simulink model "fcs_archi"  (R2023b)
settings: Solver=FixedStepAuto  StartTime=0.0  StopTime=10.0  FixedStep=5e-5  RelTol=1e-3
InitFcn:
  | addpath('c\');
  | addpath('enums\');
values from neighbouring files (symbols this model uses):
  Climb_Alt = 50.0    [fcs_spec.sldd]
  density_of_air = 1.2    [fcs_spec.sldd]
  f_Baro_Alt = 50.0    [fcs_spec.sldd]
  f_fidr = 400.0    [fcs_spec.sldd]
  f_GPS = 10.0    [fcs_spec.sldd]
  f_IMU = 800.0    [fcs_spec.sldd]
  f_inner_loop = 400.0    [fcs_spec.sldd]
  f_Mag = 50.0    [fcs_spec.sldd]
  f_mission_manager = 50.0    [fcs_spec.sldd]
  f_outer_loop = 50.0    [fcs_spec.sldd]
  f_Pitot = 50.0    [fcs_spec.sldd]
  f_sensor_acquisition = 400.0    [fcs_spec.sldd]
  g = 9.8    [fcs_spec.sldd]
  Pitch_Angle_Max = 0.4363    [fcs_spec.sldd]
  Pitch_Angle_Min = -0.261799    [fcs_spec.sldd]
  Pitch_Rate_Max = 1.05    [fcs_spec.sldd]
  Roll_Angle_Max = 1.15    [fcs_spec.sldd]
  Roll_Rate_Max = 1.57    [fcs_spec.sldd]
  Takeoff_Alt = 2.0    [fcs_spec.sldd]
  Takeoff_Spd = 50.0    [fcs_spec.sldd]
  Yaw_Rate_Max = 0.52    [fcs_spec.sldd]
undefined symbols (not defined in the file or in its folder): DiscIntNeverNeededParam, Sensor_Mode
libraries: dspfdesign x5, simulink x3, sharedtransform x1
(part 1 of 2)
settings Model: DataDictionary=fcs_spec.sldd  Creator=Aniket  LastModifiedBy=Aniket
settings SFSimCC: SimUserIncludeDirs=.\c
settings SFSimCC: SimCustomHeaderCode=|
  | #include "attitude_controller.h"
  | #include "pos_alt_controller.h"
settings SFSimCC: SimUserSources=|
  | attitude_controller.c
  | pos_alt_controller.c
settings ConfigComp: DVTestSuiteOptimization=Auto  DVDetectOutOfBounds=on  DVModelReferenceHarness=on  DVHarnessSource=Signal Editor  DVRebuildModelRepresentation=IfChangeIsDetected

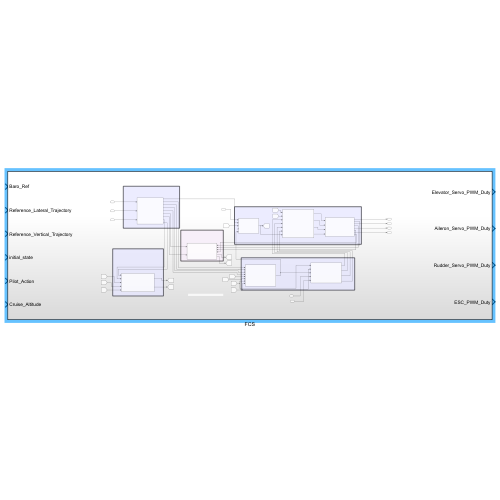
[thumbnail: Simulink's stored preview of the top-level diagram]
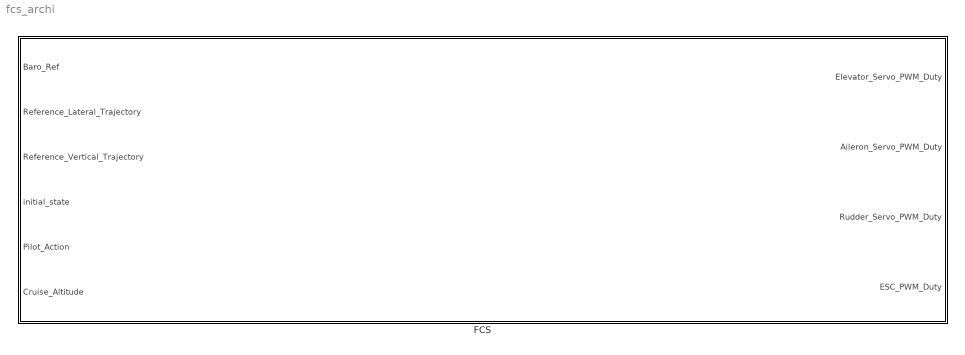
== system fcs_archi ==
  FCS : Subsystem

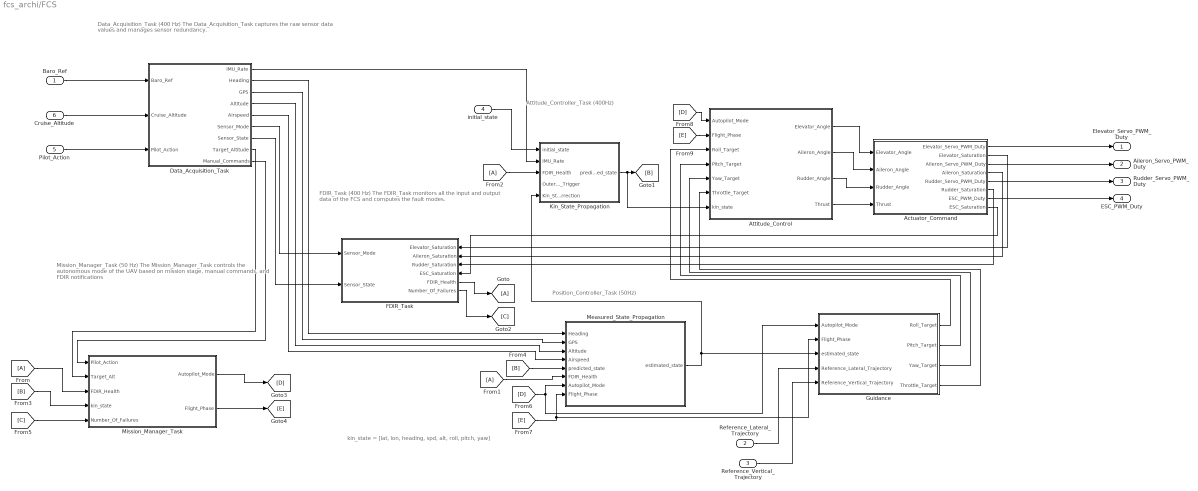
== system fcs_archi/FCS ==
  note: kin_state = [lat, lon, heading, spd, alt, roll, pitch, yaw]
  note: Mission_Manager_Task (50 Hz)
      | The Mission_Manager_Task controls the autonomous mode
      | of the UAV based on mission stage, manual commands, and
      | FDIR notifications
  note: Attitude_Controller_Task (400Hz)
  note: FDIR_Task (400 Hz)
      | The FDIR_Task monitors all the input
      | and output data of the FCS and computes the fault
      | modes.
  note: Data_Acquisition_Task (400 Hz)
      | The Data_Acquisition_Task captures the raw sensor data values
      | and manages sensor redundancy.
  note: Position_Controller_Task (50Hz)
  Baro_Ref : Inport
  Reference_Lateral_Trajectory : Inport  Port=2
  Reference_Vertical_Trajectory : Inport  Port=3
  initial_state : Inport  Port=4
  Pilot_Action : Inport  Port=5
  Cruise_Altitude : Inport  Port=6
  Actuator_Command : Subsystem
  Attitude_Control : Subsystem
  Data_Acquisition_Task : Subsystem
  FDIR_Task : Subsystem
      settings: PortSchema="{\"entries\":[{\"content\":{\"sides\":[{\"content\":{\"connectorIds\":[\"In1\",\"In2\"]},\"type\":\"ConnectorPlacement.EquallySpacedRectSide\",\"uuid\":\"991e8061-6223-401d-b3d8-a02ac305caf5\"},{\"content\":{\"connectorIds\":[\"In3\",\"In4\",\"In5\",\"In6\",\"Out1\",\"Out2\"],\"side\":\"RIGHT\"},\"type\":\"ConnectorPlacement.EquallySpacedRectSide\",\"uuid\":\"39839a1c-9529-4bba-bfe7-212855812bb8\"},{\"content\":{\"side\":\"TOP\"},\"type\":\"ConnectorPlacement.EquallySpacedRectSide\",\"uuid\":\"1450207f-9818-4db6-97f8-8e2891081434\"}]},\"type\":\"ConnectorPlacement.EquallySpacedConnector\",\"uuid\":\"30fba5ee-2c18-47f5-b9c2-5959a4a20b0d\"}],\"packageUris\":[\"http://schema.mathworks.com/mf0/Connector/R2020b\"],\"version\":\"1.0\"}"
  From : From
  From1 : From
  From2 : From
  Goto : Goto
  Guidance : Subsystem
  Kin_State_Propagation : Subsystem
  Measured_State_Propagation : Subsystem
  Mission_Manager_Task : Subsystem
  Elevator_Servo_PWM_Duty : Outport
  Aileron_Servo_PWM_Duty : Outport  Port=2
  Rudder_Servo_PWM_Duty : Outport  Port=3
  ESC_PWM_Duty : Outport  Port=4
  wires:
  Reference_Vertical_Trajectory/1 -> Guidance/5(Reference_Vertical_Trajectory)
  Data_Acquisition_Task/4(Altitude) -> Measured_State_Propagation/3(Altitude)
  Measured_State_Propagation/1(estimated_state) -> Kin_State_Propagation/5(Kin_State_correction), Guidance/3(estimated_state)
  Data_Acquisition_Task/6(Sensor_Mode) -> FDIR_Task/1(Sensor_Mode)
  Kin_State_Propagation/1(predicted_state) -> [B], Attitude_Control/7(kin_state)
  Data_Acquisition_Task/2(Heading) -> Measured_State_Propagation/1(Heading)
  Data_Acquisition_Task/3(GPS) -> Measured_State_Propagation/2(GPS)
  Actuator_Command/3(Aileron_Servo_PWM_Duty) -> Aileron_Servo_PWM_Duty/1
  Data_Acquisition_Task/7(Sensor_State) -> FDIR_Task/2(Sensor_State)
  Guidance/3(Yaw_Target) -> Attitude_Control/5(Yaw_Target)
  Data_Acquisition_Task/5(Airspeed) -> Measured_State_Propagation/4(Airspeed)
  Actuator_Command/6(Rudder_Saturation) -> FDIR_Task/5(Rudder_Saturation)
  Actuator_Command/2(Elevator_Saturation) -> FDIR_Task/3(Elevator_Saturation)
  Guidance/4(Throttle_Target) -> Attitude_Control/6(Throttle_Target)
  Data_Acquisition_Task/1(IMU_Rate) -> Kin_State_Propagation/2(IMU_Rate)
  Reference_Lateral_Trajectory/1 -> Guidance/4(Reference_Lateral_Trajectory)
  Guidance/1(Roll_Target) -> Attitude_Control/3(Roll_Target)
  Actuator_Command/5(Rudder_Servo_PWM_Duty) -> Rudder_Servo_PWM_Duty/1
  Guidance/2(Pitch_Target) -> Attitude_Control/4(Pitch_Target)
  Attitude_Control/3(Rudder_Angle) -> Actuator_Command/3(Rudder_Angle)
  Actuator_Command/4(Aileron_Saturation) -> FDIR_Task/4(Aileron_Saturation)
  Attitude_Control/1(Elevator_Angle) -> Actuator_Command/1(Elevator_Angle)
  Attitude_Control/4(Thrust) -> Actuator_Command/4(Thrust)
  Attitude_Control/2(Aileron_Angle) -> Actuator_Command/2(Aileron_Angle)
  Actuator_Command/8(ESC_Saturation) -> FDIR_Task/6(ESC_Saturation)
  Baro_Ref/1 -> Data_Acquisition_Task/1(Baro_Ref)
  Actuator_Command/1(Elevator_Servo_PWM_Duty) -> Elevator_Servo_PWM_Duty/1
  Actuator_Command/7(ESC_PWM_Duty) -> ESC_PWM_Duty/1
  initial_state/1 -> Kin_State_Propagation/1(initial_state)
  FDIR_Task/1(FDIR_Health) -> Goto/1
  From/1 -> Mission_Manager_Task/3(FDIR_Health)
  From1/1 -> Measured_State_Propagation/6(FDIR_Health)
  From2/1 -> Kin_State_Propagation/3(FDIR_Health)
  [B] -> Mission_Manager_Task/4(kin_state)
  [B] -> Measured_State_Propagation/5(predicted_state)
  Pilot_Action/1 -> Data_Acquisition_Task/3(Pilot_Action)
  FDIR_Task/2(Number_Of_Failures) -> [C]
  [C] -> Mission_Manager_Task/5(Number_Of_Failures)
  Cruise_Altitude/1 -> Data_Acquisition_Task/2(Cruise_Altitude)
  Mission_Manager_Task/1(Autopilot_Mode) -> [D]
  Mission_Manager_Task/2(Flight_Phase) -> [E]
  [D] -> Attitude_Control/1(Autopilot_Mode)
  [E] -> Attitude_Control/2(Flight_Phase)
  Data_Acquisition_Task/9(Manual_Commands) -> Mission_Manager_Task/1(Pilot_Action)
  Data_Acquisition_Task/8(Target_Altitude) -> Mission_Manager_Task/2(Target_Alt)
  [D] -> Measured_State_Propagation/7(Autopilot_Mode), Guidance/1(Autopilot_Mode)
  [E] -> Measured_State_Propagation/8(Flight_Phase), Guidance/2(Flight_Phase)

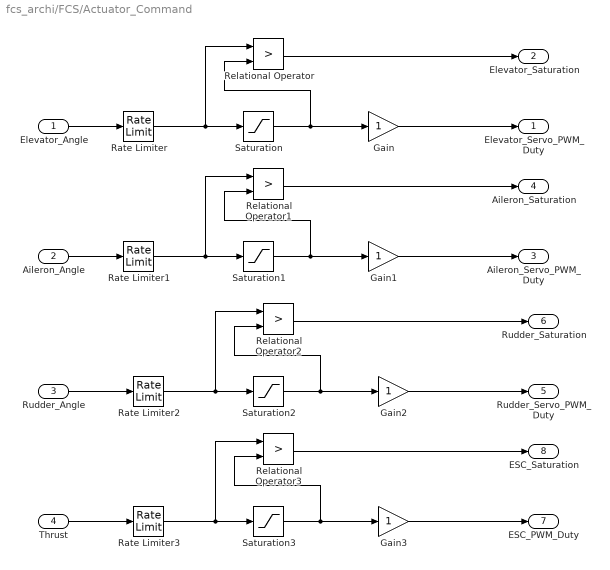
== system fcs_archi/FCS/Actuator_Command ==
  Elevator_Angle : Inport
  Aileron_Angle : Inport  Port=2
  Rudder_Angle : Inport  Port=3
  Thrust : Inport  Port=4
  Gain{,1..3} (4 alike) : Gain
  Rate Limiter{,1..3} (4 alike) : RateLimiter  SampleTimeMode=inherited
  Relational Operator{,1..3} (4 alike) : RelationalOperator  Operator=>  OutDataTypeStr=boolean  RndMeth=Simplest  InputSameDT=off
  Saturation{,1..3} (4 alike) : Saturate
  Elevator_Servo_PWM_Duty : Outport
  Elevator_Saturation : Outport  Port=2
  Aileron_Servo_PWM_Duty : Outport  Port=3
  Aileron_Saturation : Outport  Port=4
  Rudder_Servo_PWM_Duty : Outport  Port=5
  Rudder_Saturation : Outport  Port=6
  ESC_PWM_Duty : Outport  Port=7
  ESC_Saturation : Outport  Port=8
  wires:
  Elevator_Angle/1 -> Rate Limiter/1
  Rate Limiter/1 -> Relational Operator/1, Saturation/1
  Saturation/1 -> Relational Operator/2, Gain/1
  Gain/1 -> Elevator_Servo_PWM_Duty/1
  Relational Operator/1 -> Elevator_Saturation/1
  Relational Operator1/1 -> Aileron_Saturation/1
  Rate Limiter1/1 -> Relational Operator1/1, Saturation1/1
  Gain1/1 -> Aileron_Servo_PWM_Duty/1
  Saturation1/1 -> Relational Operator1/2, Gain1/1
  Aileron_Angle/1 -> Rate Limiter1/1
  Relational Operator2/1 -> Rudder_Saturation/1
  Saturation3/1 -> Relational Operator3/2, Gain3/1
  Rate Limiter3/1 -> Relational Operator3/1, Saturation3/1
  Relational Operator3/1 -> ESC_Saturation/1
  Gain3/1 -> ESC_PWM_Duty/1
  Rate Limiter2/1 -> Relational Operator2/1, Saturation2/1
  Gain2/1 -> Rudder_Servo_PWM_Duty/1
  Saturation2/1 -> Relational Operator2/2, Gain2/1
  Rudder_Angle/1 -> Rate Limiter2/1
  Thrust/1 -> Rate Limiter3/1

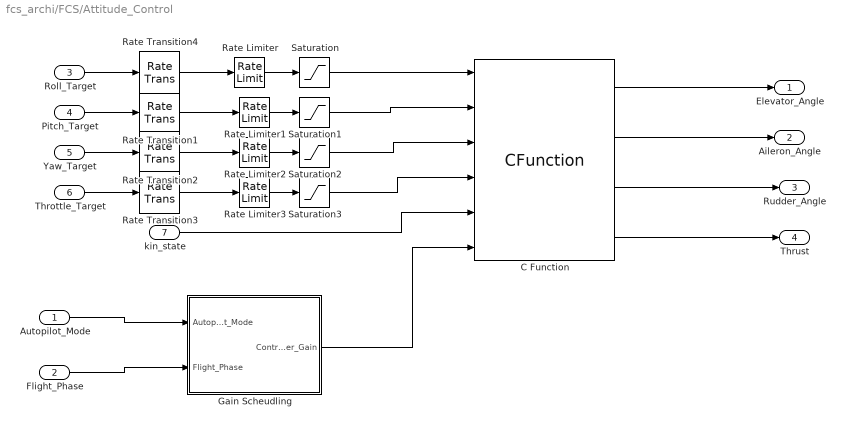
== system fcs_archi/FCS/Attitude_Control ==
  Autopilot_Mode : Inport
  Flight_Phase : Inport  Port=2
  Roll_Target : Inport  Port=3
  Pitch_Target : Inport  Port=4
  Yaw_Target : Inport  Port=5
  Throttle_Target : Inport  Port=6
  kin_state : Inport  Port=7
  C Function : CFunction  OutputCode=compute(Gain, Roll_Target, Pitch_Target, Yaw_Target, Throttle_Target, kin_state, &Elevator_Angle, &Aileron_Angle, &Rudder_Angle, &Thrust);
  Gain Scheudling : Subsystem  TreatAsAtomicUnit=on
  Rate Limiter{,1..3} (4 alike) : RateLimiter  SampleTimeMode=inherited
  Rate Transition{1..4} (4 alike) : RateTransition  OutPortSampleTime=1/f_inner_loop
  Saturation{,1..3} (4 alike) : Saturate
  Elevator_Angle : Outport
  Aileron_Angle : Outport  Port=2
  Rudder_Angle : Outport  Port=3
  Thrust : Outport  Port=4
  wires:
  Roll_Target/1 -> Rate Transition4/1
  Pitch_Target/1 -> Rate Transition1/1
  Yaw_Target/1 -> Rate Transition2/1
  Throttle_Target/1 -> Rate Transition3/1
  Rate Limiter/1 -> Saturation/1
  Saturation/1 -> C Function/1
  Rate Limiter1/1 -> Saturation1/1
  Saturation1/1 -> C Function/2
  Rate Limiter2/1 -> Saturation2/1
  Saturation2/1 -> C Function/3
  Rate Limiter3/1 -> Saturation3/1
  Saturation3/1 -> C Function/4
  kin_state/1 -> C Function/5
  C Function/1 -> Elevator_Angle/1
  C Function/2 -> Aileron_Angle/1
  C Function/3 -> Rudder_Angle/1
  C Function/4 -> Thrust/1
  Rate Transition4/1 -> Rate Limiter/1
  Rate Transition1/1 -> Rate Limiter1/1
  Rate Transition3/1 -> Rate Limiter3/1
  Rate Transition2/1 -> Rate Limiter2/1
  Autopilot_Mode/1 -> Gain Scheudling/1(Autopilot_Mode)
  Flight_Phase/1 -> Gain Scheudling/2(Flight_Phase)
  Gain Scheudling/1(Controller_Gain) -> C Function/6

== system fcs_archi/FCS/Data_Acquisition_Task ==
  Baro_Ref : Inport
  Cruise_Altitude : Inport  Port=2
  Pilot_Action : Inport  Port=3
  Data_Acquisition : Subsystem
  Measurement : Subsystem
  IMU_Rate : Outport
  Heading : Outport  Port=2
  GPS : Outport  Port=3
  Altitude : Outport  Port=4
  Airspeed : Outport  Port=5
  Sensor_Mode : Outport  Port=6
  Sensor_State : Outport  Port=7
  Target_Altitude : Outport  Port=8
  Manual_Commands : Outport  Port=9
  wires:
  Data_Acquisition/1(IMU_Mean) -> Measurement/1(IMU_Mean)
  Data_Acquisition/2(Mag_Mean) -> Measurement/2(Mag_Mean)
  Data_Acquisition/3(GPS_Mean) -> Measurement/3(GPS_Mean)
  Data_Acquisition/4(Baro_Alt_Mean) -> Measurement/4(Baro_Alt_Mean)
  Data_Acquisition/5(Pitot_Mean) -> Measurement/5(Pitot_Mean)
  Data_Acquisition/6(Mode) -> Sensor_Mode/1
  Data_Acquisition/7(Sensor_State) -> Sensor_State/1
  Baro_Ref/1 -> Measurement/6(Baro_Ref)
  Measurement/1(IMU_Rate) -> IMU_Rate/1
  Measurement/3(GPS) -> GPS/1
  Measurement/2(Heading) -> Heading/1
  Measurement/5(Airspeed) -> Airspeed/1
  Measurement/4(Altitude) -> Altitude/1
  Cruise_Altitude/1 -> Data_Acquisition/1(Cruise_Altitude_Raw)
  Pilot_Action/1 -> Data_Acquisition/2(Pilot_Action_Raw)
  Data_Acquisition/8(Cruise_Altitude) -> Target_Altitude/1
  Data_Acquisition/9(Pilot_Action) -> Manual_Commands/1

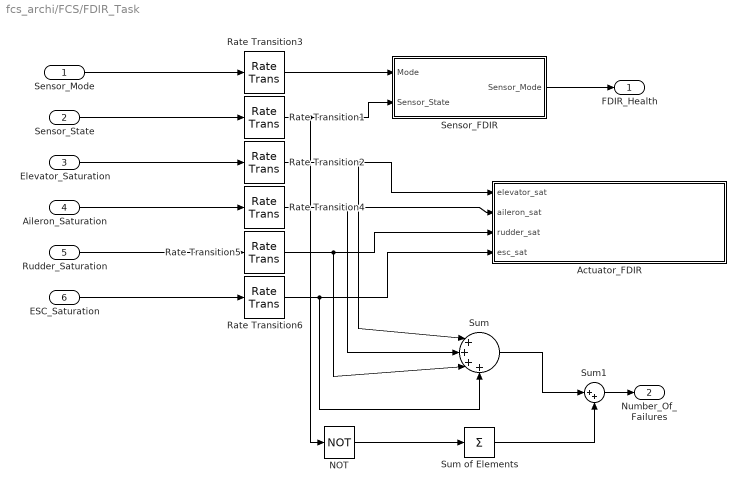
== system fcs_archi/FCS/FDIR_Task ==
  Sensor_Mode : Inport  OutDataTypeStr=Enum: Sensor_Mode
  Sensor_State : Inport  Port=2
  Elevator_Saturation : Inport  Port=3
  Aileron_Saturation : Inport  Port=4
  Rudder_Saturation : Inport  Port=5
  ESC_Saturation : Inport  Port=6
  Actuator_FDIR : MATLAB Function  TreatAsAtomicUnit=on
  NOT : Logic  Operator=NOT  IconShape=distinctive  AllPortsSameDT=off  OutDataTypeStr=boolean
  Rate Transition{1..6} (6 alike) : RateTransition  OutPortSampleTime=1/f_fidr
  Sensor_FDIR : Subsystem
  Sum : Sum  Inputs=|++++
  Sum of Elements : Sum  Inputs=+
  Sum1 : Sum  Inputs=|++
  FDIR_Health : Outport
  Number_Of_Failures : Outport  Port=2
  wires:
  Sensor_Mode/1 -> Rate Transition3/1
  Sensor_State/1 -> Rate Transition1/1
  Sensor_FDIR/1(Sensor_Mode) -> FDIR_Health/1
  Rate Transition3/1 -> Sensor_FDIR/1(Mode)
  Rate Transition1/1 -> NOT/1, Sensor_FDIR/2(Sensor_State)
  Elevator_Saturation/1 -> Rate Transition2/1
  Aileron_Saturation/1 -> Rate Transition4/1
  Rudder_Saturation/1 -> Rate Transition5/1
  ESC_Saturation/1 -> Rate Transition6/1
  Rate Transition2/1 -> Actuator_FDIR/1(elevator_sat), Sum/1
  Rate Transition4/1 -> Actuator_FDIR/2(aileron_sat), Sum/2
  Rate Transition5/1 -> Sum/3, Actuator_FDIR/3(rudder_sat)
  Rate Transition6/1 -> Actuator_FDIR/4(esc_sat), Sum/4
  NOT/1 -> Sum of Elements/1
  Sum/1 -> Sum1/1
  Sum of Elements/1 -> Sum1/2
  Sum1/1 -> Number_Of_Failures/1

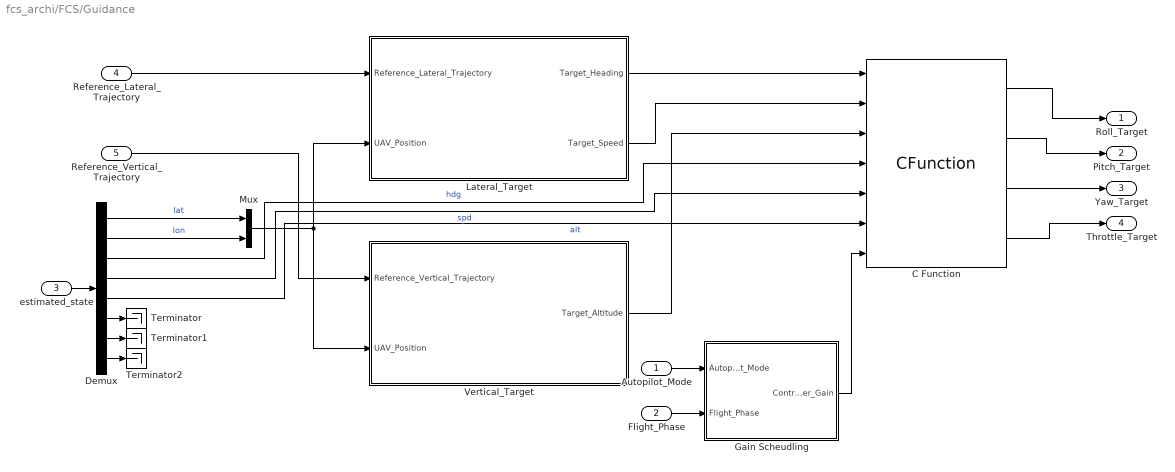
== system fcs_archi/FCS/Guidance ==
  Autopilot_Mode : Inport
  Flight_Phase : Inport  Port=2
  estimated_state : Inport  Port=3
  Reference_Lateral_Trajectory : Inport  Port=4
  Reference_Vertical_Trajectory : Inport  Port=5
  C Function : CFunction  OutputCode=compute_targets(Gain, Target_Hdg, Target_Spd, Target_Alt, Estimated_Hdg, Estimated_Spd, Estimated_Alt, &Roll_Target, &Pitch_Target, &Yaw_Target, &Throttle_Target);
  Demux : Demux  Outputs=8
  Gain Scheudling : Subsystem  TreatAsAtomicUnit=on
  Lateral_Target : Subsystem
  Mux : Mux  Inputs=2
  Terminator : Terminator
  Terminator1 : Terminator
  Terminator2 : Terminator
  Vertical_Target : Subsystem
  Roll_Target : Outport
  Pitch_Target : Outport  Port=2
  Yaw_Target : Outport  Port=3
  Throttle_Target : Outport  Port=4
  wires:
  Reference_Lateral_Trajectory/1 -> Lateral_Target/1(Reference_Lateral_Trajectory)
  estimated_state/1 -> Demux/1
  Demux/1 -> Mux/1  "lat"
  Demux/2 -> Mux/2  "lon"
  Mux/1 -> Vertical_Target/2(UAV_Position), Lateral_Target/2(UAV_Position)
  Reference_Vertical_Trajectory/1 -> Vertical_Target/1(Reference_Vertical_Trajectory)
  Lateral_Target/1(Target_Heading) -> C Function/1
  Lateral_Target/2(Target_Speed) -> C Function/2
  Vertical_Target/1(Target_Altitude) -> C Function/3
  Demux/3 -> C Function/4  "hdg"
  Demux/4 -> C Function/5  "spd"
  Demux/5 -> C Function/6  "alt"
  Demux/6 -> Terminator/1
  Demux/7 -> Terminator1/1
  Demux/8 -> Terminator2/1
  C Function/1 -> Roll_Target/1
  C Function/2 -> Pitch_Target/1
  C Function/3 -> Yaw_Target/1
  C Function/4 -> Throttle_Target/1
  Flight_Phase/1 -> Gain Scheudling/2(Flight_Phase)
  Autopilot_Mode/1 -> Gain Scheudling/1(Autopilot_Mode)
  Gain Scheudling/1(Controller_Gain) -> C Function/7

== system fcs_archi/FCS/Kin_State_Propagation ==
  initial_state : Inport
  IMU_Rate : Inport  Port=2
  FDIR_Health : Inport  Port=3
  Outer_Loop_Trigger : Inport  Port=4
  Kin_State_correction : Inport  Port=5
  "Kin_State2UAV_State " : Subsystem
  Kinematics_Propagator : Subsystem
  Mux : Mux  Inputs=8
  Rate Transition1 : RateTransition  OutPortSampleTime=1/f_inner_loop
  Rate Transition3 : RateTransition  OutPortSampleTime=1/f_inner_loop
  Rate Transition4 : RateTransition  OutPortSampleTime=1/f_inner_loop
  Switch : Switch  Criteria=u2 > Threshold  SaturateOnIntegerOverflow=off  InputSameDT=off
  UAV kinematics : Subsystem
  predicted_state : Outport
  wires:
  Kinematics_Propagator/1(dstate) -> UAV kinematics/2(dstate)
  UAV kinematics/1(state) -> Kinematics_Propagator/3(prev_state), "Kin_State2UAV_State "/1(state)  "Prediction"
  "Kin_State2UAV_State "/7(pitch) -> Mux/7
  "Kin_State2UAV_State "/2(lon) -> Mux/2
  "Kin_State2UAV_State "/4(speed) -> Mux/4
  "Kin_State2UAV_State "/3(heading) -> Mux/3
  "Kin_State2UAV_State "/5(altitude) -> Mux/5
  "Kin_State2UAV_State "/8(yaw) -> Mux/8
  FDIR_Health/1 -> Rate Transition1/1
  "Kin_State2UAV_State "/1(lat) -> Mux/1
  "Kin_State2UAV_State "/6(roll) -> Mux/6
  IMU_Rate/1 -> Rate Transition3/1
  Mux/1 -> Switch/3
  Kin_State_correction/1 -> Rate Transition4/1
  Rate Transition3/1 -> Kinematics_Propagator/1(IMU_Rate)
  Rate Transition1/1 -> Kinematics_Propagator/2(FDIR_Health)
  initial_state/1 -> UAV kinematics/1(initial_state)
  Outer_Loop_Trigger/1 -> Switch/2
  Rate Transition4/1 -> Switch/1
  Switch/1 -> predicted_state/1

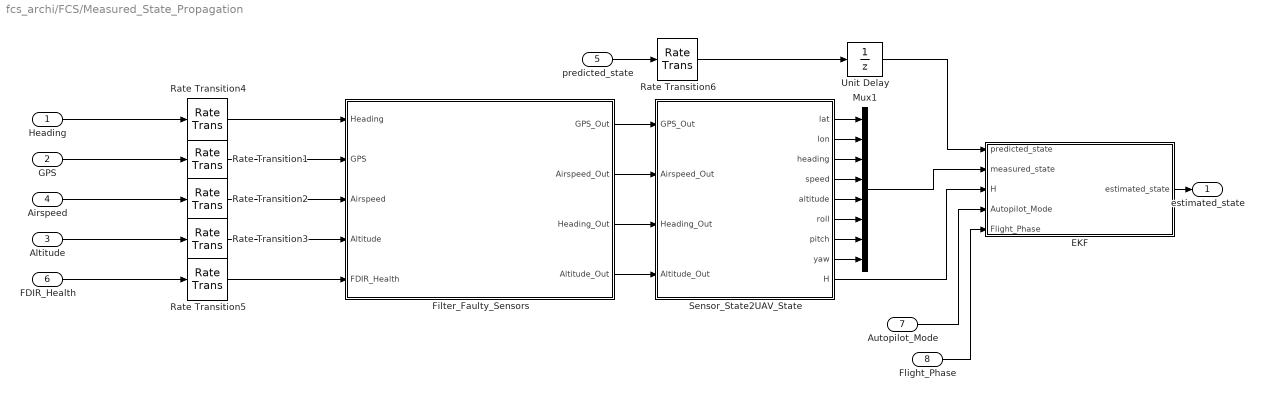
== system fcs_archi/FCS/Measured_State_Propagation ==
  Heading : Inport
  GPS : Inport  Port=2
  Altitude : Inport  Port=3
  Airspeed : Inport  Port=4
  predicted_state : Inport  Port=5
  FDIR_Health : Inport  Port=6
  Autopilot_Mode : Inport  Port=7
  Flight_Phase : Inport  Port=8
  EKF : Subsystem
  Filter_Faulty_Sensors : Subsystem
  Mux1 : Mux  Inputs=8
  Rate Transition{1..5} (5 alike) : RateTransition  OutPortSampleTime=1/f_outer_loop
  Rate Transition6 : RateTransition  OutPortSampleTime=1/f_inner_loop
  Sensor_State2UAV_State : Subsystem
  Unit Delay : UnitDelay  SampleTime=-1  HasFrameUpgradeWarning=on
  estimated_state : Outport
  wires:
  FDIR_Health/1 -> Rate Transition5/1
  Mux1/1 -> EKF/2(measured_state)
  Sensor_State2UAV_State/2(lon) -> Mux1/2
  Airspeed/1 -> Rate Transition2/1
  Sensor_State2UAV_State/1(lat) -> Mux1/1
  predicted_state/1 -> Rate Transition6/1
  EKF/1(estimated_state) -> estimated_state/1
  Filter_Faulty_Sensors/1(GPS_Out) -> Sensor_State2UAV_State/1(GPS_Out)
  Filter_Faulty_Sensors/2(Airspeed_Out) -> Sensor_State2UAV_State/2(Airspeed_Out)
  Filter_Faulty_Sensors/4(Altitude_Out) -> Sensor_State2UAV_State/4(Altitude_Out)
  Altitude/1 -> Rate Transition3/1
  Filter_Faulty_Sensors/3(Heading_Out) -> Sensor_State2UAV_State/3(Heading_Out)
  Sensor_State2UAV_State/9(H) -> EKF/3(H)
  GPS/1 -> Rate Transition1/1
  Heading/1 -> Rate Transition4/1
  Sensor_State2UAV_State/3(heading) -> Mux1/3
  Sensor_State2UAV_State/4(speed) -> Mux1/4
  Sensor_State2UAV_State/5(altitude) -> Mux1/5
  Sensor_State2UAV_State/6(roll) -> Mux1/6
  Sensor_State2UAV_State/7(pitch) -> Mux1/7
  Sensor_State2UAV_State/8(yaw) -> Mux1/8
  Rate Transition4/1 -> Filter_Faulty_Sensors/1(Heading)
  Rate Transition1/1 -> Filter_Faulty_Sensors/2(GPS)
  Rate Transition2/1 -> Filter_Faulty_Sensors/3(Airspeed)
  Rate Transition5/1 -> Filter_Faulty_Sensors/5(FDIR_Health)
  Rate Transition3/1 -> Filter_Faulty_Sensors/4(Altitude)
  Rate Transition6/1 -> Unit Delay/1
  Unit Delay/1 -> EKF/1(predicted_state)
  Autopilot_Mode/1 -> EKF/4(Autopilot_Mode)
  Flight_Phase/1 -> EKF/5(Flight_Phase)

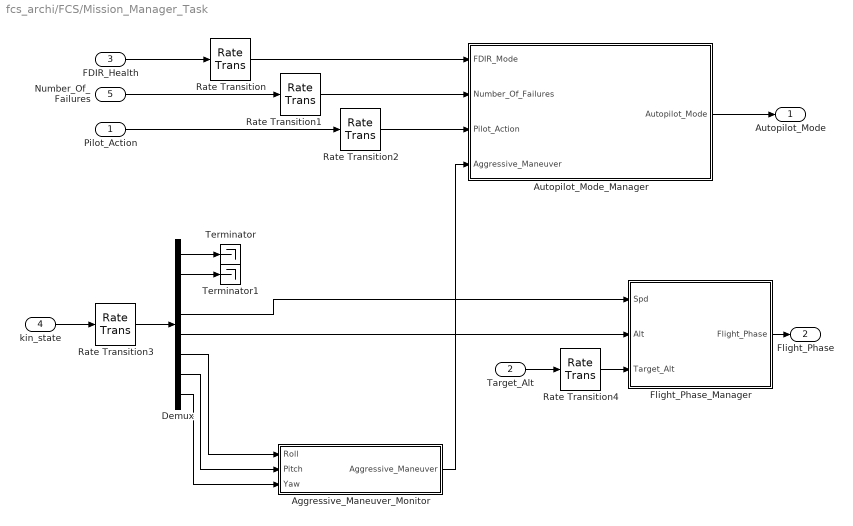
== system fcs_archi/FCS/Mission_Manager_Task ==
  Pilot_Action : Inport
  Target_Alt : Inport  Port=2
  FDIR_Health : Inport  Port=3
  kin_state : Inport  Port=4
  Number_Of_Failures : Inport  Port=5
  Aggressive_Maneuver_Monitor : Subsystem
  Autopilot_Mode_Manager : Stateflow chart  TreatAsAtomicUnit=on
  Demux : Demux  Outputs=8
  Flight_Phase_Manager : Stateflow chart  TreatAsAtomicUnit=on
  Rate Transition{,1..4} (5 alike) : RateTransition  OutPortSampleTime=1/f_mission_manager
  Terminator : Terminator
  Terminator1 : Terminator
  Autopilot_Mode : Outport
  Flight_Phase : Outport  Port=2
  wires:
  kin_state/1 -> Rate Transition3/1
  Target_Alt/1 -> Rate Transition4/1
  Demux/4 -> Flight_Phase_Manager/1(Spd)
  Demux/5 -> Flight_Phase_Manager/2(Alt)
  Demux/1 -> Terminator/1
  Demux/2 -> Terminator1/1
  Demux/6 -> Aggressive_Maneuver_Monitor/1(Roll)
  Demux/7 -> Aggressive_Maneuver_Monitor/2(Pitch)
  Demux/8 -> Aggressive_Maneuver_Monitor/3(Yaw)
  Number_Of_Failures/1 -> Rate Transition1/1
  FDIR_Health/1 -> Rate Transition/1
  Pilot_Action/1 -> Rate Transition2/1
  Autopilot_Mode_Manager/1(Autopilot_Mode) -> Autopilot_Mode/1
  Flight_Phase_Manager/1(Flight_Phase) -> Flight_Phase/1
  Aggressive_Maneuver_Monitor/1(Aggressive_Maneuver) -> Autopilot_Mode_Manager/4(Aggressive_Maneuver)
  Rate Transition/1 -> Autopilot_Mode_Manager/1(FDIR_Mode)
  Rate Transition1/1 -> Autopilot_Mode_Manager/2(Number_Of_Failures)
  Rate Transition2/1 -> Autopilot_Mode_Manager/3(Pilot_Action)
  Rate Transition3/1 -> Demux/1
  Rate Transition4/1 -> Flight_Phase_Manager/3(Target_Alt)

== system fcs_archi/FCS/Attitude_Control/Gain Scheudling ==
  Autopilot_Mode : Inport
  Flight_Phase : Inport  Port=2
  Controller_Gain : Outport

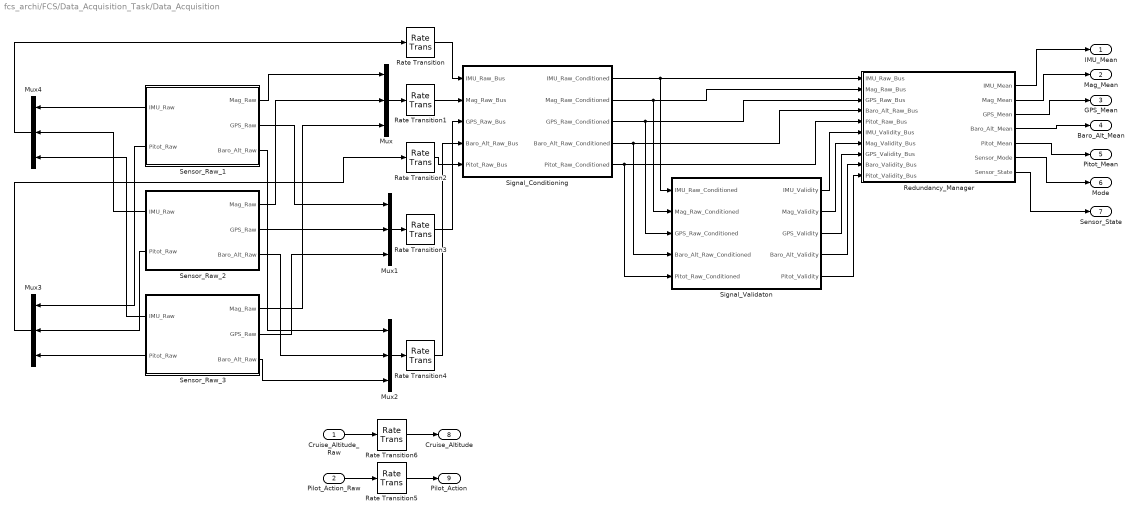
== system fcs_archi/FCS/Data_Acquisition_Task/Data_Acquisition ==
  Cruise_Altitude_Raw : Inport
  Pilot_Action_Raw : Inport  Port=2
  Mux{,1..4} (5 alike) : Mux  Inputs=3
  Rate Transition{,1..6} (7 alike) : RateTransition  OutPortSampleTime=1/f_sensor_acquisition
  Redundancy_Manager : Subsystem
  Sensor_Raw_1 : Subsystem
      settings: PortSchema="{\"entries\":[{\"content\":{\"sides\":[{\"content\":{\"connectorIds\":[\"Out4\",\"Out5\"]},\"type\":\"ConnectorPlacement.EquallySpacedRectSide\",\"uuid\":\"715424aa-37ae-40bf-9508-94e341e62c8d\"},{\"content\":{\"connectorIds\":[\"Out1\",\"Out2\",\"Out3\"],\"side\":\"RIGHT\"},\"type\":\"ConnectorPlacement.EquallySpacedRectSide\",\"uuid\":\"e53a2a69-e3e6-44f0-8b80-70a275b8a431\"},{\"content\":{\"side\":\"TOP\"},\"type\":\"ConnectorPlacement.EquallySpacedRectSide\",\"uuid\":\"55883ea8-dd36-4c27-8de9-fa1a8e6b43b3\"}]},\"type\":\"ConnectorPlacement.EquallySpacedConnector\",\"uuid\":\"0d9dd66d-5cf8-423e-9621-2547ec94f36a\"}],\"packageUris\":[\"http://schema.mathworks.com/mf0/Connector/R2020b\"],\"version\":\"1.0\"}"
  Sensor_Raw_2 : Subsystem
      settings: PortSchema="{\"entries\":[{\"content\":{\"sides\":[{\"content\":{\"connectorIds\":[\"Out4\",\"Out5\"]},\"type\":\"ConnectorPlacement.EquallySpacedRectSide\",\"uuid\":\"715424aa-37ae-40bf-9508-94e341e62c8d\"},{\"content\":{\"connectorIds\":[\"Out1\",\"Out2\",\"Out3\"],\"side\":\"RIGHT\"},\"type\":\"ConnectorPlacement.EquallySpacedRectSide\",\"uuid\":\"e53a2a69-e3e6-44f0-8b80-70a275b8a431\"},{\"content\":{\"side\":\"TOP\"},\"type\":\"ConnectorPlacement.EquallySpacedRectSide\",\"uuid\":\"55883ea8-dd36-4c27-8de9-fa1a8e6b43b3\"}]},\"type\":\"ConnectorPlacement.EquallySpacedConnector\",\"uuid\":\"0d9dd66d-5cf8-423e-9621-2547ec94f36a\"}],\"packageUris\":[\"http://schema.mathworks.com/mf0/Connector/R2020b\"],\"version\":\"1.0\"}"
  Sensor_Raw_3 : Subsystem
      settings: PortSchema="{\"entries\":[{\"content\":{\"sides\":[{\"content\":{\"connectorIds\":[\"Out4\",\"Out5\"]},\"type\":\"ConnectorPlacement.EquallySpacedRectSide\",\"uuid\":\"715424aa-37ae-40bf-9508-94e341e62c8d\"},{\"content\":{\"connectorIds\":[\"Out1\",\"Out2\",\"Out3\"],\"side\":\"RIGHT\"},\"type\":\"ConnectorPlacement.EquallySpacedRectSide\",\"uuid\":\"e53a2a69-e3e6-44f0-8b80-70a275b8a431\"},{\"content\":{\"side\":\"TOP\"},\"type\":\"ConnectorPlacement.EquallySpacedRectSide\",\"uuid\":\"55883ea8-dd36-4c27-8de9-fa1a8e6b43b3\"}]},\"type\":\"ConnectorPlacement.EquallySpacedConnector\",\"uuid\":\"0d9dd66d-5cf8-423e-9621-2547ec94f36a\"}],\"packageUris\":[\"http://schema.mathworks.com/mf0/Connector/R2020b\"],\"version\":\"1.0\"}"
  Signal_Conditioning : Subsystem
  Signal_Validaton : Subsystem
  IMU_Mean : Outport
  Mag_Mean : Outport  Port=2
  GPS_Mean : Outport  Port=3
  Baro_Alt_Mean : Outport  Port=4
  Pitot_Mean : Outport  Port=5
  Mode : Outport  Port=6
  Sensor_State : Outport  Port=7
  Cruise_Altitude : Outport  Port=8
  Pilot_Action : Outport  Port=9
  wires:
  Sensor_Raw_2/4(IMU_Raw) -> Mux4/2
  Sensor_Raw_2/2(GPS_Raw) -> Mux1/2
  Sensor_Raw_1/1(Mag_Raw) -> Mux/1
  Sensor_Raw_3/3(Baro_Alt_Raw) -> Mux2/3
  Sensor_Raw_1/4(IMU_Raw) -> Mux4/1
  Sensor_Raw_3/1(Mag_Raw) -> Mux/3
  Mux2/1 -> Rate Transition4/1
  Sensor_Raw_2/1(Mag_Raw) -> Mux/2
  Mux4/1 -> Rate Transition/1
  Sensor_Raw_2/5(Pitot_Raw) -> Mux3/2
  Sensor_Raw_1/2(GPS_Raw) -> Mux1/1
  Sensor_Raw_2/3(Baro_Alt_Raw) -> Mux2/2
  Sensor_Raw_1/3(Baro_Alt_Raw) -> Mux2/1
  Sensor_Raw_3/4(IMU_Raw) -> Mux4/3
  Mux/1 -> Rate Transition1/1
  Mux1/1 -> Rate Transition3/1
  Sensor_Raw_1/5(Pitot_Raw) -> Mux3/1
  Sensor_Raw_3/5(Pitot_Raw) -> Mux3/3
  Sensor_Raw_3/2(GPS_Raw) -> Mux1/3
  Mux3/1 -> Rate Transition2/1
  Redundancy_Manager/1(IMU_Mean) -> IMU_Mean/1
  Redundancy_Manager/2(Mag_Mean) -> Mag_Mean/1
  Redundancy_Manager/7(Sensor_State) -> Sensor_State/1
  Redundancy_Manager/4(Baro_Alt_Mean) -> Baro_Alt_Mean/1
  Redundancy_Manager/3(GPS_Mean) -> GPS_Mean/1
  Redundancy_Manager/5(Pitot_Mean) -> Pitot_Mean/1
  Redundancy_Manager/6(Sensor_Mode) -> Mode/1
  Signal_Conditioning/1(IMU_Raw_Conditioned) -> Signal_Validaton/1(IMU_Raw_Conditioned), Redundancy_Manager/1(IMU_Raw_Bus)
  Signal_Conditioning/2(Mag_Raw_Conditioned) -> Signal_Validaton/2(Mag_Raw_Conditioned), Redundancy_Manager/2(Mag_Raw_Bus)
  Signal_Conditioning/3(GPS_Raw_Conditioned) -> Signal_Validaton/3(GPS_Raw_Conditioned), Redundancy_Manager/3(GPS_Raw_Bus)
  Signal_Conditioning/4(Baro_Alt_Raw_Conditioned) -> Redundancy_Manager/4(Baro_Alt_Raw_Bus), Signal_Validaton/4(Baro_Alt_Raw_Conditioned)
  Signal_Conditioning/5(Pitot_Raw_Conditioned) -> Redundancy_Manager/5(Pitot_Raw_Bus), Signal_Validaton/5(Pitot_Raw_Conditioned)
  Signal_Validaton/1(IMU_Validity) -> Redundancy_Manager/6(IMU_Validity_Bus)
  Signal_Validaton/2(Mag_Validity) -> Redundancy_Manager/7(Mag_Validity_Bus)
  Signal_Validaton/3(GPS_Validity) -> Redundancy_Manager/8(GPS_Validity_Bus)
  Signal_Validaton/4(Baro_Alt_Validity) -> Redundancy_Manager/9(Baro_Validity_Bus)
  Signal_Validaton/5(Pitot_Validity) -> Redundancy_Manager/10(Pitot_Validity_Bus)
  Rate Transition/1 -> Signal_Conditioning/1(IMU_Raw_Bus)
  Rate Transition1/1 -> Signal_Conditioning/2(Mag_Raw_Bus)
  Rate Transition2/1 -> Signal_Conditioning/5(Pitot_Raw_Bus)
  Rate Transition3/1 -> Signal_Conditioning/3(GPS_Raw_Bus)
  Rate Transition4/1 -> Signal_Conditioning/4(Baro_Alt_Raw_Bus)
  Cruise_Altitude_Raw/1 -> Rate Transition6/1
  Pilot_Action_Raw/1 -> Rate Transition5/1
  Rate Transition6/1 -> Cruise_Altitude/1
  Rate Transition5/1 -> Pilot_Action/1

== system fcs_archi/FCS/Data_Acquisition_Task/Measurement ==
  IMU_Mean : Inport
  Mag_Mean : Inport  Port=2
  GPS_Mean : Inport  Port=3
  Baro_Alt_Mean : Inport  Port=4
  Pitot_Mean : Inport  Port=5
  Baro_Ref : Inport  Port=6
  Convert_Baro_To_Alt : Subsystem
  Convert_Mag_Declination_To_Heading : Subsystem
  Convert_Pressure_To_Airspeed : Subsystem
  Sum : Sum  Inputs=|+-
  Unit Delay : UnitDelay  SampleTime=-1  HasFrameUpgradeWarning=on
  IMU_Rate : Outport
  Heading : Outport  Port=2
  GPS : Outport  Port=3
  Altitude : Outport  Port=4
  Airspeed : Outport  Port=5
  wires:
  Mag_Mean/1 -> Convert_Mag_Declination_To_Heading/1(Mag_Mean)
  Baro_Alt_Mean/1 -> Sum/1
  Baro_Ref/1 -> Sum/2
  GPS_Mean/1 -> GPS/1
  Sum/1 -> Convert_Baro_To_Alt/1(Pressure)
  Convert_Baro_To_Alt/1(Altitude) -> Convert_Pressure_To_Airspeed/2(Altitude), Unit Delay/1, Altitude/1
  Unit Delay/1 -> Convert_Baro_To_Alt/2(Prev_Altitude)
  Pitot_Mean/1 -> Convert_Pressure_To_Airspeed/1(Pressure)
  Convert_Pressure_To_Airspeed/1(Airspeed) -> Airspeed/1
  IMU_Mean/1 -> IMU_Rate/1
  Convert_Mag_Declination_To_Heading/1(Mag_Heading) -> Heading/1

== system fcs_archi/FCS/FDIR_Task/Sensor_FDIR ==
  Mode : Inport
  Sensor_State : Inport  Port=2
  Demux : Demux  Outputs=5
  Measurement_Health : Stateflow chart  TreatAsAtomicUnit=on
  Notify_D1 : Stateflow chart  TreatAsAtomicUnit=on
      settings: PortSchema="{\"entries\":[{\"content\":{\"sides\":[{\"content\":{\"connectorIds\":[\"In1\",\"In3\",\"In5\",\"In2\",\"In4\"]},\"type\":\"ConnectorPlacement.EquallySpacedRectSide\",\"uuid\":\"1c3396b1-7836-4a39-8c87-e624726558fd\"},{\"content\":{\"connectorIds\":[\"Out1\"],\"side\":\"RIGHT\"},\"type\":\"ConnectorPlacement.EquallySpacedRectSide\",\"uuid\":\"729d4963-88fb-4f29-94e7-d92fa754ed0a\"},{\"content\":{\"side\":\"TOP\"},\"type\":\"ConnectorPlacement.EquallySpacedRectSide\",\"uuid\":\"14efdf31-8350-4a5c-bb6e-ff3a1bfbe15c\"}]},\"type\":\"ConnectorPlacement.EquallySpacedConnector\",\"uuid\":\"cda37305-181d-4b82-bf72-7af95c41c2d1\"}],\"packageUris\":[\"http://schema.mathworks.com/mf0/Connector/R2020b\"],\"version\":\"1.0\"}"
  Notify_D1_Sensor_State : Subsystem  TreatAsAtomicUnit=on
  Notify_D2_Sensor_State : Subsystem  TreatAsAtomicUnit=on
  Switch Case : SwitchCase  CaseConditions={Sensor_FDIR_Mode('No_IMU_GPS')}
  Terminator : Terminator
  Sensor_Mode : Outport
  wires:
  Switch Case/2 -> Terminator/1
  Demux/2 -> Notify_D1/3(Mag_Mode), Measurement_Health/3(Mag_Mode)
  Demux/3 -> Notify_D1/5(GPS_Mode), Measurement_Health/5(GPS_Mode)
  Demux/4 -> Notify_D1/2(Baro_Alt_Mode), Measurement_Health/2(Baro_Alt_Mode)
  Measurement_Health/1(Sensor_Mode) -> Sensor_Mode/1, Switch Case/1
  Sensor_State/1 -> Notify_D2_Sensor_State/1(Sensor_State), Notify_D1_Sensor_State/1(Sensor_State)
  Demux/1 -> Notify_D1/1(IMU_Mode), Measurement_Health/1(IMU_Mode)
  Switch Case/1 -> Notify_D2_Sensor_State/Action
  Demux/5 -> Notify_D1/4(Pitot_Mode), Measurement_Health/4(Pitot_Mode)
  Notify_D1/1(Notify_D1) -> Notify_D1_Sensor_State/Enable
  Mode/1 -> Demux/1

== system fcs_archi/FCS/Guidance/Gain Scheudling ==
  Autopilot_Mode : Inport
  Flight_Phase : Inport  Port=2
  Controller_Gain : Outport

== system fcs_archi/FCS/Guidance/Lateral_Target ==
  Reference_Lateral_Trajectory : Inport
  UAV_Position : Inport  Port=2
  Target_Heading : Outport
  Target_Speed : Outport  Port=2

== system fcs_archi/FCS/Guidance/Vertical_Target ==
  Reference_Vertical_Trajectory : Inport
  UAV_Position : Inport  Port=2
  Target_Altitude : Outport

== system fcs_archi/FCS/Kin_State_Propagation/Kin_State2UAV_State  ==
  state : Inport
  lat : Outport
  lon : Outport  Port=2
  heading : Outport  Port=3
  speed : Outport  Port=4
  altitude : Outport  Port=5
  roll : Outport  Port=6
  pitch : Outport  Port=7
  yaw : Outport  Port=8

== system fcs_archi/FCS/Kin_State_Propagation/Kinematics_Propagator ==
  IMU_Rate : Inport
  FDIR_Health : Inport  Port=2
  prev_state : Inport  Port=3
  If Action Subsystem : Subsystem  TreatAsAtomicUnit=on
  Merge : Merge
  Switch Case : SwitchCase  CaseConditions={[Sensor_FDIR_Mode('No_IMU_GPS'), Sensor_FDIR_Mode('No_IMU')]}
  UAV dynamics : Subsystem  TreatAsAtomicUnit=on
  dstate : Outport
  wires:
  FDIR_Health/1 -> Switch Case/1
  Switch Case/2 -> If Action Subsystem/Action
  IMU_Rate/1 -> If Action Subsystem/1(IMU_Rate)
  If Action Subsystem/1(dstate) -> Merge/1
  Merge/1 -> dstate/1
  Switch Case/1 -> UAV dynamics/Action
  UAV dynamics/1(dstate) -> Merge/2
  prev_state/1 -> UAV dynamics/1(state)

== system fcs_archi/FCS/Kin_State_Propagation/UAV kinematics ==
  note: kinematic_state = [x,y,z,roll,pitch,yaw]
  initial_state : Inport
  dstate : Inport  Port=2
  Demux : Demux  Outputs=2
  Demux1 : Demux  Outputs=2
  Demux2 : Demux  Outputs=3
  Discrete-Time Integrator : DiscreteIntegrator  InitialConditionSource=external  SampleTime=-1  ICPrevOutput=DiscIntNeverNeededParam  ICPrevScaledInput=DiscIntNeverNeededParam
  MATLAB Function : MATLAB Function  TreatAsAtomicUnit=on
  Mux1 : Mux  Inputs=2
  Product : Product  Multiplication=Matrix(*)
  Rotation Angles to Direction Cosine Matrix : sharedtransform/Rotation Angles to Direction Cosine Matrix  rotationOrder=ZYX  aMode=aMode
  Terminator : Terminator
  Terminator1 : Terminator
  state : Outport
  wires:
  dstate/1 -> Demux/1
  MATLAB Function/1(euler_angle_rate) -> Mux1/2
  initial_state/1 -> Discrete-Time Integrator/2
  Demux/2 -> MATLAB Function/1(w)
  Demux/1 -> Product/2
  Demux2/1 -> MATLAB Function/2(roll)
  Demux2/2 -> MATLAB Function/3(pitch)
  Discrete-Time Integrator/1 -> Demux1/1, state/1
  Demux2/3 -> Terminator/1
  Rotation Angles to Direction Cosine Matrix/1 -> Product/1
  Product/1 -> Mux1/1
  Mux1/1 -> Discrete-Time Integrator/1
  Demux1/2 -> Demux2/1, Rotation Angles to Direction Cosine Matrix/1
  Demux1/1 -> Terminator1/1

== system fcs_archi/FCS/Measured_State_Propagation/EKF ==
  predicted_state : Inport
  measured_state : Inport  Port=2
  H : Inport  Port=3
  Autopilot_Mode : Inport  Port=4
  Flight_Phase : Inport  Port=5
  estimated_state : Outport
  wires:
  predicted_state/1 -> estimated_state/1

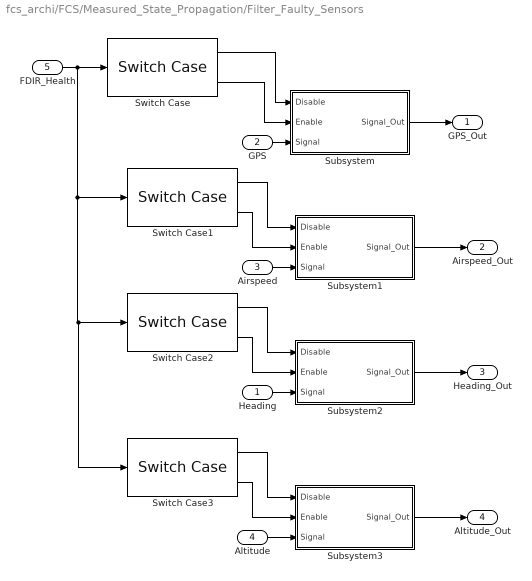
== system fcs_archi/FCS/Measured_State_Propagation/Filter_Faulty_Sensors ==
  Heading : Inport
  GPS : Inport  Port=2
  Airspeed : Inport  Port=3
  Altitude : Inport  Port=4
  FDIR_Health : Inport  Port=5
  Subsystem : Subsystem
  Subsystem1 : Subsystem
  Subsystem2 : Subsystem
  Subsystem3 : Subsystem
  Switch Case : SwitchCase  CaseConditions={[Sensor_FDIR_Mode('No_IMU_GPS'),Sensor_FDIR_Mode('No_GPS')]}
  Switch Case1 : SwitchCase  CaseConditions={[Sensor_FDIR_Mode('No_IMU_GPS'),Sensor_FDIR_Mode('No_IMU'),Sensor_FDIR_Mode('GPS_Spd'),Sensor_FDIR_Mode('GPS_Alt_Spd'),Sensor_FDIR_Mode('GPS_Spd_Hdg')]}
  Switch Case2 : SwitchCase  CaseConditions={[Sensor_FDIR_Mode('No_IMU_GPS'),Sensor_FDIR_Mode('No_IMU'),Sensor_FDIR_Mode('GPS_Hdg'),Sensor_FDIR_Mode('GPS_Spd_Hdg'),Sensor_FDIR_Mode('GPS_Alt_Hdg')]}
  Switch Case3 : SwitchCase  CaseConditions={[Sensor_FDIR_Mode('No_IMU_GPS'),Sensor_FDIR_Mode('No_IMU'),Sensor_FDIR_Mode('GPS_Alt'),Sensor_FDIR_Mode('GPS_Alt_Spd'),Sensor_FDIR_Mode('GPS_Alt_Hdg')]}
  GPS_Out : Outport
  Airspeed_Out : Outport  Port=2
  Heading_Out : Outport  Port=3
  Altitude_Out : Outport  Port=4
  wires:
  Switch Case/1 -> Subsystem/1(Disable)
  Switch Case/2 -> Subsystem/2(Enable)
  GPS/1 -> Subsystem/3(Signal)
  Subsystem/1(Signal_Out) -> GPS_Out/1
  Airspeed/1 -> Subsystem1/3(Signal)
  Subsystem1/1(Signal_Out) -> Airspeed_Out/1
  Switch Case1/1 -> Subsystem1/1(Disable)
  Switch Case1/2 -> Subsystem1/2(Enable)
  Heading/1 -> Subsystem2/3(Signal)
  Switch Case2/2 -> Subsystem2/2(Enable)
  Switch Case2/1 -> Subsystem2/1(Disable)
  Subsystem2/1(Signal_Out) -> Heading_Out/1
  Altitude/1 -> Subsystem3/3(Signal)
  FDIR_Health/1 -> Switch Case3/1, Switch Case2/1, Switch Case1/1, Switch Case/1
  Switch Case3/1 -> Subsystem3/1(Disable)
  Subsystem3/1(Signal_Out) -> Altitude_Out/1
  Switch Case3/2 -> Subsystem3/2(Enable)

== system fcs_archi/FCS/Measured_State_Propagation/Sensor_State2UAV_State ==
  note: Dummy_Implementation
      |
      | Logic needs to be implemented to pick the sensor fusion quantities based on quality of the data (Airspeed from pitot tube is more preferable than GPS speed when both are available) and filter out the NaN signals
      |
      | Entries of H matrix for measurement equation can be made zero to not consider them for measurement update
  GPS_Out : Inport
  Airspeed_Out : Inport  Port=2
  Heading_Out : Inport  Port=3
  Altitude_Out : Inport  Port=4
  lat : Outport
  lon : Outport  Port=2
  heading : Outport  Port=3
  speed : Outport  Port=4
  altitude : Outport  Port=5
  roll : Outport  Port=6
  pitch : Outport  Port=7
  yaw : Outport  Port=8
  H : Outport  Port=9

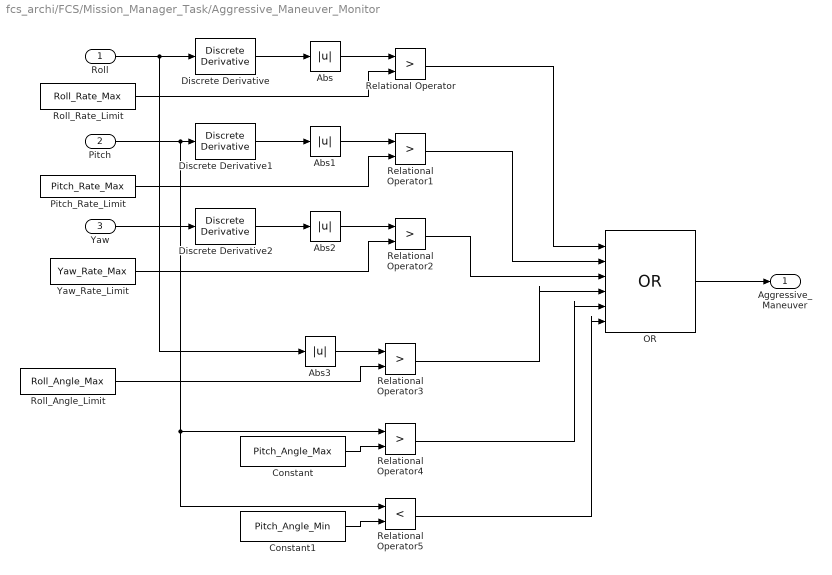
== system fcs_archi/FCS/Mission_Manager_Task/Aggressive_Maneuver_Monitor ==
  Roll : Inport
  Pitch : Inport  Port=2
  Yaw : Inport  Port=3
  Abs{,1..3} (4 alike) : Abs  SaturateOnIntegerOverflow=off
  Constant : Constant  Value=Pitch_Angle_Max
  Constant1 : Constant  Value=Pitch_Angle_Min
  Discrete Derivative : simulink/Discrete/Discrete Derivative  gainval=1.0  ICPrevScaledInput=0.0  OutMin=[]  OutMax=[]  OutDataType=fixdt(1, 16)  OutScaling=2^-10  DoSatur=off
  Discrete Derivative1 : simulink/Discrete/Discrete Derivative  gainval=1.0  ICPrevScaledInput=0.0  OutMin=[]  OutMax=[]  OutDataType=fixdt(1, 16)  OutScaling=2^-10  DoSatur=off
  Discrete Derivative2 : simulink/Discrete/Discrete Derivative  gainval=1.0  ICPrevScaledInput=0.0  OutMin=[]  OutMax=[]  OutDataType=fixdt(1, 16)  OutScaling=2^-10  DoSatur=off
  OR : Logic  Operator=OR  Inputs=6  IconShape=distinctive  AllPortsSameDT=off  OutDataTypeStr=boolean
  Pitch_Rate_Limit : Constant  Value=Pitch_Rate_Max
  Relational Operator{,1..4} (5 alike) : RelationalOperator  Operator=>  OutDataTypeStr=boolean  RndMeth=Simplest  InputSameDT=off
  Relational Operator5 : RelationalOperator  Operator=<  OutDataTypeStr=boolean  RndMeth=Simplest  InputSameDT=off
  Roll_Angle_Limit : Constant  Value=Roll_Angle_Max
  Roll_Rate_Limit : Constant  Value=Roll_Rate_Max
  Yaw_Rate_Limit : Constant  Value=Yaw_Rate_Max
  Aggressive_Maneuver : Outport
  wires:
  Roll/1 -> Abs3/1, Discrete Derivative/1
  Pitch/1 -> Discrete Derivative1/1, Relational Operator5/1, Relational Operator4/1
  Yaw/1 -> Discrete Derivative2/1
  Discrete Derivative/1 -> Abs/1
  Discrete Derivative1/1 -> Abs1/1
  Discrete Derivative2/1 -> Abs2/1
  Abs/1 -> Relational Operator/1
  Abs1/1 -> Relational Operator1/1
  Abs2/1 -> Relational Operator2/1
  Roll_Rate_Limit/1 -> Relational Operator/2
  Relational Operator/1 -> OR/1
  Relational Operator1/1 -> OR/2
  Relational Operator2/1 -> OR/3
  Pitch_Rate_Limit/1 -> Relational Operator1/2
  Yaw_Rate_Limit/1 -> Relational Operator2/2
  Abs3/1 -> Relational Operator3/1
  Roll_Angle_Limit/1 -> Relational Operator3/2
  Constant/1 -> Relational Operator4/2
  Constant1/1 -> Relational Operator5/2
  Relational Operator3/1 -> OR/4
  Relational Operator4/1 -> OR/5
  Relational Operator5/1 -> OR/6
  OR/1 -> Aggressive_Maneuver/1

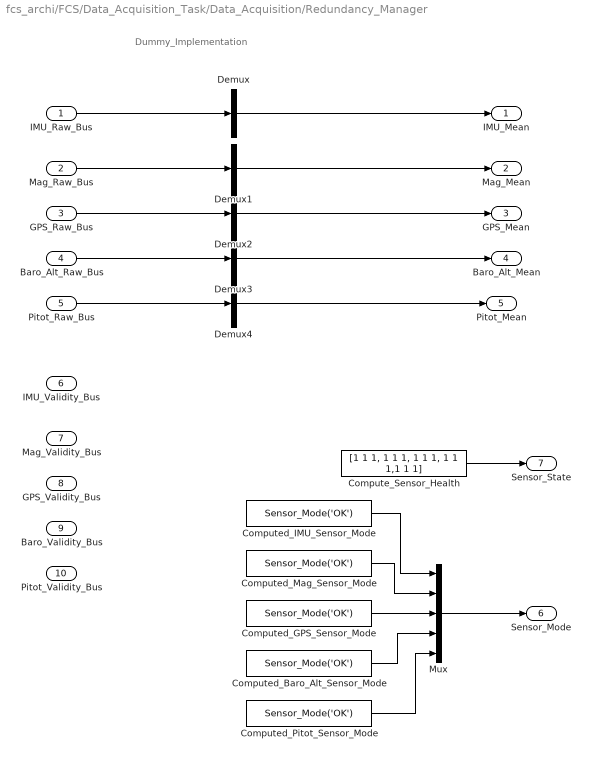
== system fcs_archi/FCS/Data_Acquisition_Task/Data_Acquisition/Redundancy_Manager ==
  note: Dummy_Implementation
  IMU_Raw_Bus : Inport
  Mag_Raw_Bus : Inport  Port=2
  GPS_Raw_Bus : Inport  Port=3
  Baro_Alt_Raw_Bus : Inport  Port=4
  Pitot_Raw_Bus : Inport  Port=5
  IMU_Validity_Bus : Inport  Port=6
  Mag_Validity_Bus : Inport  Port=7
  GPS_Validity_Bus : Inport  Port=8
  Baro_Validity_Bus : Inport  Port=9
  Pitot_Validity_Bus : Inport  Port=10
  Compute_Sensor_Health : Constant  Value=[1 1 1, 1 1 1, 1 1 1, 1 1 1,1 1 1]
  Computed_Baro_Alt_Sensor_Mode : Constant  Value=Sensor_Mode('OK')  OutDataTypeStr=Enum: Sensor_Mode
  Computed_GPS_Sensor_Mode : Constant  Value=Sensor_Mode('OK')  OutDataTypeStr=Enum: Sensor_Mode
  Computed_IMU_Sensor_Mode : Constant  Value=Sensor_Mode('OK')  OutDataTypeStr=Enum: Sensor_Mode
  Computed_Mag_Sensor_Mode : Constant  Value=Sensor_Mode('OK')  OutDataTypeStr=Enum: Sensor_Mode
  Computed_Pitot_Sensor_Mode : Constant  Value=Sensor_Mode('OK')  OutDataTypeStr=Enum: Sensor_Mode
  Demux{,1..4} (5 alike) : Demux  Outputs=3
  Mux : Mux  Inputs=5
  IMU_Mean : Outport
  Mag_Mean : Outport  Port=2
  GPS_Mean : Outport  Port=3
  Baro_Alt_Mean : Outport  Port=4
  Pitot_Mean : Outport  Port=5
  Sensor_Mode : Outport  Port=6
  Sensor_State : Outport  Port=7
  wires:
  IMU_Raw_Bus/1 -> Demux/1
  Mag_Raw_Bus/1 -> Demux1/1
  Demux/2 -> IMU_Mean/1
  Demux1/2 -> Mag_Mean/1
  GPS_Raw_Bus/1 -> Demux2/1
  Demux2/2 -> GPS_Mean/1
  Baro_Alt_Raw_Bus/1 -> Demux3/1
  Demux3/2 -> Baro_Alt_Mean/1
  Pitot_Raw_Bus/1 -> Demux4/1
  Demux4/2 -> Pitot_Mean/1
  Compute_Sensor_Health/1 -> Sensor_State/1
  Mux/1 -> Sensor_Mode/1
  Computed_Mag_Sensor_Mode/1 -> Mux/2
  Computed_Baro_Alt_Sensor_Mode/1 -> Mux/4
  Computed_Pitot_Sensor_Mode/1 -> Mux/5
  Computed_GPS_Sensor_Mode/1 -> Mux/3
  Computed_IMU_Sensor_Mode/1 -> Mux/1

== system fcs_archi/FCS/Data_Acquisition_Task/Data_Acquisition/Sensor_Raw_1 ==
  Baro_Alt : Constant  Value=ones(1,1)  SampleTime=1/f_Baro_Alt
  GPS : Constant  Value=ones(5,1)  SampleTime=1/f_GPS
  IMU : Constant  Value=ones(6,1)  SampleTime=1/f_IMU
  Mag : Constant  Value=ones(3,1)  SampleTime=1/f_Mag
  Pitot : Constant  Value=ones(1,1)  SampleTime=1/f_Pitot
  Mag_Raw : Outport
  GPS_Raw : Outport  Port=2
  Baro_Alt_Raw : Outport  Port=3
  IMU_Raw : Outport  Port=4
  Pitot_Raw : Outport  Port=5
  wires:
  IMU/1 -> IMU_Raw/1
  Mag/1 -> Mag_Raw/1
  Baro_Alt/1 -> Baro_Alt_Raw/1
  GPS/1 -> GPS_Raw/1
  Pitot/1 -> Pitot_Raw/1

== system fcs_archi/FCS/Data_Acquisition_Task/Data_Acquisition/Sensor_Raw_2 ==
  Baro_Alt : Constant  Value=ones(1,1)
  GPS : Constant  Value=ones(5,1)
  IMU : Constant  Value=ones(6,1)
  Mag : Constant  Value=ones(3,1)
  Pitot : Constant  Value=ones(1,1)
  Mag_Raw : Outport
  GPS_Raw : Outport  Port=2
  Baro_Alt_Raw : Outport  Port=3
  IMU_Raw : Outport  Port=4
  Pitot_Raw : Outport  Port=5
  wires:
  IMU/1 -> IMU_Raw/1
  Mag/1 -> Mag_Raw/1
  Baro_Alt/1 -> Baro_Alt_Raw/1
  GPS/1 -> GPS_Raw/1
  Pitot/1 -> Pitot_Raw/1

== system fcs_archi/FCS/Data_Acquisition_Task/Data_Acquisition/Sensor_Raw_3 ==
  Baro_Alt : Constant  Value=ones(1,1)
  GPS : Constant  Value=ones(5,1)
  IMU : Constant  Value=ones(6,1)
  Mag : Constant  Value=ones(3,1)
  Pitot : Constant  Value=ones(1,1)
  Mag_Raw : Outport
  GPS_Raw : Outport  Port=2
  Baro_Alt_Raw : Outport  Port=3
  IMU_Raw : Outport  Port=4
  Pitot_Raw : Outport  Port=5
  wires:
  IMU/1 -> IMU_Raw/1
  Mag/1 -> Mag_Raw/1
  Baro_Alt/1 -> Baro_Alt_Raw/1
  GPS/1 -> GPS_Raw/1
  Pitot/1 -> Pitot_Raw/1

== system fcs_archi/FCS/Data_Acquisition_Task/Data_Acquisition/Signal_Conditioning ==
  IMU_Raw_Bus : Inport
  Mag_Raw_Bus : Inport  Port=2
  GPS_Raw_Bus : Inport  Port=3
  Baro_Alt_Raw_Bus : Inport  Port=4
  Pitot_Raw_Bus : Inport  Port=5
  Lowpass Filter{,1..4} (5 alike) : dspfdesign/Lowpass Filter  FilterType=FIR  DesignForMinimumOrder=on  FilterOrder=50  PassbandFrequency=8e3  StopbandFrequency=12e3  PassbandRipple=0.1  StopbandAttenuation=80  SampleRateMode=Specify on dialog  SampleRate=44100  SimulateUsing=Interpreted execution  roundingMode=Floor  coeffsDataTypeStr=fixdt(1,16)
  IMU_Raw_Conditioned : Outport
  Mag_Raw_Conditioned : Outport  Port=2
  GPS_Raw_Conditioned : Outport  Port=3
  Baro_Alt_Raw_Conditioned : Outport  Port=4
  Pitot_Raw_Conditioned : Outport  Port=5
  wires:
  Mag_Raw_Bus/1 -> Lowpass Filter1/1
  IMU_Raw_Bus/1 -> Lowpass Filter/1
  Baro_Alt_Raw_Bus/1 -> Lowpass Filter3/1
  GPS_Raw_Bus/1 -> Lowpass Filter2/1
  Pitot_Raw_Bus/1 -> Lowpass Filter4/1
  Lowpass Filter/1 -> IMU_Raw_Conditioned/1
  Lowpass Filter1/1 -> Mag_Raw_Conditioned/1
  Lowpass Filter2/1 -> GPS_Raw_Conditioned/1
  Lowpass Filter3/1 -> Baro_Alt_Raw_Conditioned/1
  Lowpass Filter4/1 -> Pitot_Raw_Conditioned/1

== system fcs_archi/FCS/Data_Acquisition_Task/Data_Acquisition/Signal_Validaton ==
  IMU_Raw_Conditioned : Inport
  Mag_Raw_Conditioned : Inport  Port=2
  GPS_Raw_Conditioned : Inport  Port=3
  Baro_Alt_Raw_Conditioned : Inport  Port=4
  Pitot_Raw_Conditioned : Inport  Port=5
  Dummy_Max : Constant  Value=1e3
  Dummy_Min : Constant  Value=-1e3
  Subsystem : Subsystem
  Subsystem1 : Subsystem
  Subsystem2 : Subsystem
  Subsystem3 : Subsystem
  Subsystem4 : Subsystem
  IMU_Validity : Outport
  Mag_Validity : Outport  Port=2
  GPS_Validity : Outport  Port=3
  Baro_Alt_Validity : Outport  Port=4
  Pitot_Validity : Outport  Port=5
  wires:
  Mag_Raw_Conditioned/1 -> Subsystem1/2(Signal)
  Baro_Alt_Raw_Conditioned/1 -> Subsystem3/2(Signal)
  GPS_Raw_Conditioned/1 -> Subsystem2/2(Signal)
  Pitot_Raw_Conditioned/1 -> Subsystem4/2(Signal)
  Subsystem3/1(Validity) -> Baro_Alt_Validity/1
  Subsystem4/1(Validity) -> Pitot_Validity/1
  IMU_Raw_Conditioned/1 -> Subsystem/2(Signal)
  Subsystem/1(Validity) -> IMU_Validity/1
  Subsystem1/1(Validity) -> Mag_Validity/1
  Subsystem2/1(Validity) -> GPS_Validity/1
  Dummy_Max/1 -> Subsystem1/1(Max), Subsystem4/1(Max), Subsystem3/1(Max), Subsystem2/1(Max), Subsystem/1(Max)
  Dummy_Min/1 -> Subsystem/3(Min), Subsystem4/3(Min), Subsystem3/3(Min), Subsystem2/3(Min), Subsystem1/3(Min)

== system fcs_archi/FCS/Data_Acquisition_Task/Measurement/Convert_Baro_To_Alt ==
  note: Altitude is used to calculate density of air using Standard Atmospheric Model
  note: Dummy_Implementation
  Pressure : Inport
  Prev_Altitude : Inport  Port=2
  Gain : Gain  Gain=1/(density_of_air*g)
  Terminator : Terminator
  Altitude : Outport
  wires:
  Pressure/1 -> Gain/1
  Prev_Altitude/1 -> Terminator/1
  Gain/1 -> Altitude/1

== system fcs_archi/FCS/Data_Acquisition_Task/Measurement/Convert_Mag_Declination_To_Heading ==
  note: Dummy_Implementation
  Mag_Mean : Inport
  Gain : Gain  Gain=1/3*[1 1 1]  Multiplication=Matrix(K*u)
  Mag_Heading : Outport
  wires:
  Mag_Mean/1 -> Gain/1
  Gain/1 -> Mag_Heading/1

== system fcs_archi/FCS/Data_Acquisition_Task/Measurement/Convert_Pressure_To_Airspeed ==
  note: Altitude is used to calculate density of air using Standard Atmospheric Model
  note: Dummy_Implementation
  Pressure : Inport
  Altitude : Inport  Port=2
  Gain : Gain  Gain=2/density_of_air
  Sqrt : Sqrt
  Terminator : Terminator
  Airspeed : Outport
  wires:
  Pressure/1 -> Gain/1
  Gain/1 -> Sqrt/1
  Altitude/1 -> Terminator/1
  Sqrt/1 -> Airspeed/1

== system fcs_archi/FCS/FDIR_Task/Sensor_FDIR/Notify_D1_Sensor_State ==
  Sensor_State : Inport
  Enable : EnablePort
  notify_D1 : MATLAB Function  TreatAsAtomicUnit=on
  wires:
  Sensor_State/1 -> notify_D1/1(sensor_state)

== system fcs_archi/FCS/FDIR_Task/Sensor_FDIR/Notify_D2_Sensor_State ==
  Sensor_State : Inport
  Action Port : ActionPort  ActionPortLabel=case [ No_IMU_GPS ]:
  notify_D2 : MATLAB Function  TreatAsAtomicUnit=on
  wires:
  Sensor_State/1 -> notify_D2/1(sensor_state)

== system fcs_archi/FCS/Kin_State_Propagation/Kinematics_Propagator/If Action Subsystem ==
  IMU_Rate : Inport
  Action Port : ActionPort  ActionPortLabel=default:
  dstate : Outport
  wires:
  IMU_Rate/1 -> dstate/1

== system fcs_archi/FCS/Kin_State_Propagation/Kinematics_Propagator/UAV dynamics ==
  state : Inport
  Action Port : ActionPort  ActionPortLabel=case [ No_IMU_GPS No_IMU ]:
  UAV dynamics : Subsystem
  dstate : Outport
  wires:
  state/1 -> UAV dynamics/1(In1)
  UAV dynamics/1(Out1) -> dstate/1

== system fcs_archi/FCS/Measured_State_Propagation/Filter_Faulty_Sensors/Subsystem ==
  Disable : Inport
  Enable : Inport  Port=2
  Signal : Inport  Port=3
  Is_Available : Subsystem  TreatAsAtomicUnit=on
  Is_Not_Available : Subsystem  TreatAsAtomicUnit=on
  Merge : Merge
  NaN : Constant  Value=NaN*ones(5,1)  OutDataTypeStr=Inherit: Inherit via back propagation
  Signal_Out : Outport
  wires:
  Is_Available/1(Out1) -> Merge/1
  Is_Not_Available/1(Out1) -> Merge/2
  NaN/1 -> Is_Not_Available/1(Signal)
  Merge/1 -> Signal_Out/1
  Enable/1 -> Is_Available/Action
  Signal/1 -> Is_Available/1(Signal)
  Disable/1 -> Is_Not_Available/Action

== system fcs_archi/FCS/Measured_State_Propagation/Filter_Faulty_Sensors/Subsystem1 ==
  Disable : Inport
  Enable : Inport  Port=2
  Signal : Inport  Port=3
  Is_Available : Subsystem  TreatAsAtomicUnit=on
  Is_Not_Available : Subsystem  TreatAsAtomicUnit=on
  Merge : Merge
  NaN : Constant  Value=NaN  OutDataTypeStr=Inherit: Inherit via back propagation
  Signal_Out : Outport
  wires:
  Is_Available/1(Out1) -> Merge/1
  Is_Not_Available/1(Out1) -> Merge/2
  NaN/1 -> Is_Not_Available/1(Signal)
  Merge/1 -> Signal_Out/1
  Enable/1 -> Is_Available/Action
  Signal/1 -> Is_Available/1(Signal)
  Disable/1 -> Is_Not_Available/Action

== system fcs_archi/FCS/Measured_State_Propagation/Filter_Faulty_Sensors/Subsystem2 ==
  Disable : Inport
  Enable : Inport  Port=2
  Signal : Inport  Port=3
  Is_Available : Subsystem  TreatAsAtomicUnit=on
  Is_Not_Available : Subsystem  TreatAsAtomicUnit=on
  Merge : Merge
  NaN : Constant  Value=NaN  OutDataTypeStr=Inherit: Inherit via back propagation
  Signal_Out : Outport
  wires:
  Is_Available/1(Out1) -> Merge/1
  Is_Not_Available/1(Out1) -> Merge/2
  NaN/1 -> Is_Not_Available/1(Signal)
  Merge/1 -> Signal_Out/1
  Enable/1 -> Is_Available/Action
  Signal/1 -> Is_Available/1(Signal)
  Disable/1 -> Is_Not_Available/Action
